simulink model "new_algorithm_real"  (R2023b)
settings: Solver=FixedStepAuto  StartTime=0.0  StopTime=10.0  RelTol=1e-3  EnableMultiTasking=on
undefined symbols (not defined in the file): hw
libraries: raspberrypiAVlib x3, matrix_library x2, dspadpt3 x1
settings Model: SimulationMode=external  ExtModeTrigDuration=2  Creator=mykni  LastModifiedBy=mykni
settings SolverCC: PositivePriorityOrder=on
settings OptimizationCC: EnhancedBackFolding=on  PassReuseOutputArgsAs=Individual arguments  ZeroExternalMemoryAtStartup=off  ZeroInternalMemoryAtStartup=off  MaxStackSize=64  OptimizeBlockOrder=speed  DifferentSizesBufferReuse=on  OptimizationCustomize=off  EfficientTunableParamExpr=on
settings DebuggingCC: ParameterTunabilityLossMsg=error
settings HardwareCC: ProdBitPerPointer=32  ProdBitPerSizeT=32  ProdBitPerPtrDiffT=32  ProdLargestAtomicInteger=Long  ProdLargestAtomicFloat=Double  ProdWordSize=32  ProdLongLongMode=on  ProdHWDeviceType=ARM Compatible->ARM Cortex  UseEmbeddedCoderFeatures=off  UseSimulinkCoderFeatures=off
settings RTWCC: Description=Embedded Coder  SystemTargetFile=ert.tlc  HardwareBoard=Raspberry Pi  TemplateMakefile=ert_default_tmf  RTWVerbose=off  Toolchain=GNU GCC Embedded Linux  BuildConfiguration=Faster Runs
settings CodeAppCC: ForceParamTrailComments=on  OperatorAnnotations=on  SimulinkDataObjDesc=on  SFDataObjDesc=on  MangleLength=10  InsertBlockDesc=on
settings ERTTargetCC: SupportNonInlinedSFcns=on  SupportVariableSizeSignals=on  ExtMode=on  ExtModeTransport=2  ExtModeStaticAlloc=on  ExtModeMaxTrigDuration=1000  ExtModeMexFile=ext_xcp  ExtModeMexArgs='10.26.231.231' 0 17725  ExtModeIntrfLevel=Level2 - Open  ERTSrcFileBannerTemplate=codertarget_code_template.cgt  ERTHdrFileBannerTemplate=codertarget_code_template.cgt  ERTDataSrcFileTemplate=codertarget_code_template.cgt  ERTDataHdrFileTemplate=codertarget_code_template.cgt

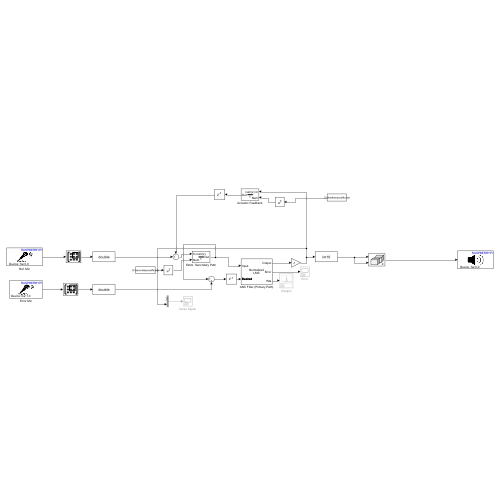
[thumbnail: Simulink's stored preview of the top-level diagram]
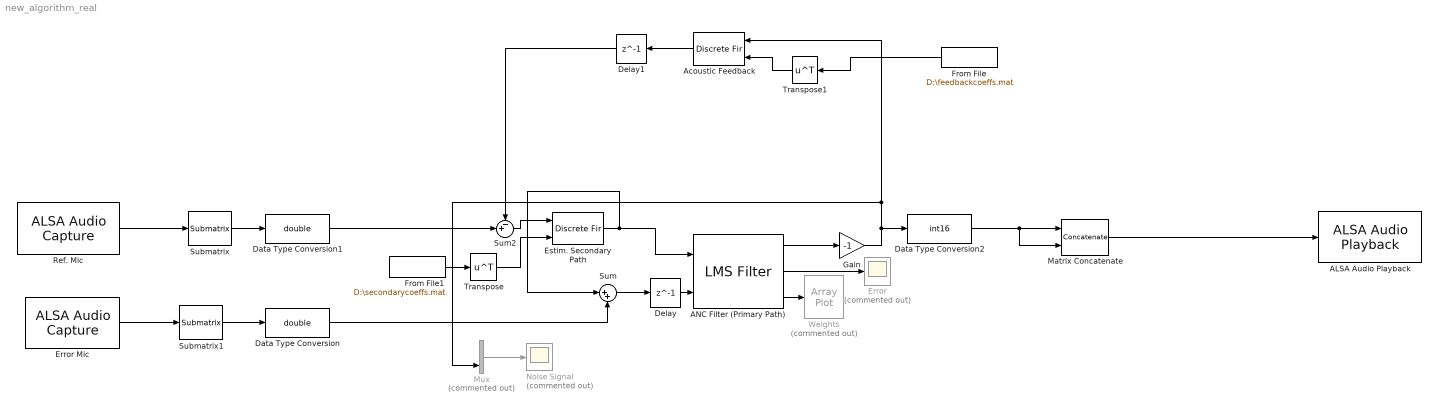
== system new_algorithm_real ==
  ALSA Audio Playback : raspberrypiAVlib/ALSA Audio Playback  deviceStr=hw:0,0  sampleRateEnum=44100  queueDuration=0.5  blockPlatform=LINUX
  ANC Filter (Primary Path) : dspadpt3/LMS Filter  Algo=Normalized LMS  L=32  stepflag=Dialog  mu=.005  leakage=1.0  ic=0  Adapt=off  resetflag=None  weights=on  addnparflag=off  roundingMode=Floor  overflowMode=off
  Acoustic Feedback : DiscreteFir  CoefSource=Input port
      settings: InputPortMap=u0,u1
  Data Type Conversion : DataTypeConversion  OutDataTypeStr=double  SaturateOnIntegerOverflow=off  RndMeth=Floor
  Data Type Conversion1 : DataTypeConversion  OutDataTypeStr=double  SaturateOnIntegerOverflow=off  RndMeth=Floor
  Data Type Conversion2 : DataTypeConversion  OutDataTypeStr=int16  SaturateOnIntegerOverflow=off  RndMeth=Floor
  Delay : Delay  DelayLength=1  InitialCondition=0
  Delay1 : Delay  DelayLength=1  InitialCondition=0
  Error : Scope  Commented=on
  Error Mic : raspberrypiAVlib/ALSA Audio Capture  deviceStr=hw:1,0  DataBitDepth=16-bit integer  numberOfChannels=2  sampleRateEnum=44100  frameSize=10  QueueDuration=0.5  blockPlatform=LINUX
  Estim. Secondary Path : DiscreteFir  CoefSource=Input port
      settings: InputPortMap=u0,u1
  From File : FromFile  FileName=D:\feedbackcoeffs.mat  SampleTime=0
  From File1 : FromFile  FileName=D:\secondarycoeffs.mat  SampleTime=0
  Gain : Gain  Gain=-1
  Matrix Concatenate : Concatenate  Mode=Multidimensional array  ConcatenateDimension=2
  Mux : Mux  Commented=on  Inputs=2
  Noise Signal : Scope  Commented=on
  Ref. Mic : raspberrypiAVlib/ALSA Audio Capture  deviceStr=hw:0,0  DataBitDepth=16-bit integer  numberOfChannels=2  sampleRateEnum=44100  frameSize=10  QueueDuration=0.5  blockPlatform=LINUX
  Submatrix : matrix_library/Submatrix  RowSpan=All rows  RowStartMode=First  RowStartIndex=1  RowEndMode=Last  RowEndIndex=1  ColSpan=One column  ColStartMode=First  ColStartIndex=1  ColEndMode=Last  ColEndIndex=1
  Submatrix1 : matrix_library/Submatrix  RowSpan=All rows  RowStartMode=First  RowStartIndex=1  RowEndMode=Last  RowEndIndex=1  ColSpan=One column  ColStartMode=First  ColStartIndex=1  ColEndMode=Last  ColEndIndex=1
  Sum : Sum  Inputs=|++
  Sum2 : Sum  Inputs=-+|
  Transpose : Math  Operator=transpose
  Transpose1 : Math  Operator=transpose
  Weights : ArrayPlot  Commented=on  WindowPosition=[368.000000,182.000000,800.000000,500.000000,]  ScopeFrameLocation=window  YLimits=[-0.0551 0.1188]
  wires:
  Estim. Secondary Path/1 -> Sum/1, ANC Filter (Primary Path)/1
  ANC Filter (Primary Path)/1 -> Gain/1
  Gain/1 -> Data Type Conversion2/1, Acoustic Feedback/1, Mux/2
  ANC Filter (Primary Path)/2 -> Error/1
  ANC Filter (Primary Path)/3 -> Weights/1
  Sum/1 -> Delay/1
  Delay/1 -> ANC Filter (Primary Path)/2
  Mux/1 -> Noise Signal/1
  Acoustic Feedback/1 -> Delay1/1
  Delay1/1 -> Sum2/1
  Sum2/1 -> Estim. Secondary Path/1
  Ref. Mic/1 -> Submatrix/1
  Error Mic/1 -> Submatrix1/1
  From File/1 -> Transpose1/1
  Transpose1/1 -> Acoustic Feedback/2
  Transpose/1 -> Estim. Secondary Path/2
  From File1/1 -> Transpose/1
  Submatrix1/1 -> Data Type Conversion/1
  Submatrix/1 -> Data Type Conversion1/1
  Matrix Concatenate/1 -> ALSA Audio Playback/1
  Data Type Conversion2/1 -> Matrix Concatenate/2, Matrix Concatenate/1
  Data Type Conversion1/1 -> Sum2/2
  Data Type Conversion/1 -> Sum/2
